simulink model "NonLinearModelWithObserver_real"  (R2022a)
settings: Solver=FixedStepAuto  StartTime=0.0  StopTime=inf  FixedStep=0.01  MaxStep=1e-3  MinStep=1e-5  RelTol=1e-3  EnableMultiTasking=on
values from neighbouring files (symbols this model uses):
  A = A_lin    [parameter_values.m]
  B = B_lin    [parameter_values.m]
  C_obs = [1 0 0 0; 0 0 1 0]    [parameter_values.m]
  K_lmi = calc_LMI_Controller(A,B,3)    [parameter_values.m]
  L = inv(P_sol)*N_sol    [calc_LMI_Observer.m]    (also in parameter_values.m = calc_LMI_Observer(A,C_obs,10))
  x0 = [deg2rad(0.1); 0; 0; 0]    [parameter_values.m]
  x_hat_0 = [0 0 0 0]    [parameter_values.m]
libraries: simulink_extras x1, svdutilitieslib x1, mbedblockslib x1
settings Model: ExtModeTrigDuration=10  Creator=schulte  LastModifiedBy=adlipke
settings SolverCC: AlgebraicLoopSolver=TrustRegion
settings DataIOCC: ReturnWorkspaceOutputs=off
settings OptimizationCC: EnhancedBackFolding=on  PassReuseOutputArgsAs=Individual arguments  ZeroExternalMemoryAtStartup=off  ZeroInternalMemoryAtStartup=off  MaxStackSize=64  OptimizeBlockOrder=speed  DifferentSizesBufferReuse=on  OptimizationCustomize=off  EfficientTunableParamExpr=on
settings DebuggingCC: ParameterTunabilityLossMsg=error  UnconnectedInputMsg=warning  UnconnectedOutputMsg=warning  UnconnectedLineMsg=warning  SFUnexpectedBacktrackingDiag=warning  SFNoUnconditionalDefaultTransitionDiag=warning  SFMachineParentedDataDiag=warning  ArithmeticOperatorsInVariantConditions=warning
settings HardwareCC: ProdBitPerPointer=32  ProdBitPerSizeT=32  ProdBitPerPtrDiffT=32  ProdLargestAtomicInteger=Long  ProdLargestAtomicFloat=Double  ProdWordSize=32  ProdLongLongMode=on  ProdHWDeviceType=ARM Compatible->ARM Cortex
settings SFSimCC: SimUseLocalCustomCode=off  MATLABDynamicMemAlloc=off  CustomCodeUndefinedFunction=UseInterfaceOnly
settings RTWCC: SystemTargetFile=ert.tlc  HardwareBoard=STM32 Nucleo L476RG  TemplateMakefile=ert_default_tmf  RTWUseLocalCustomCode=off  Toolchain=GNU Tools for ARM Embedded Processors
settings CodeAppCC: ForceParamTrailComments=on  IgnoreCustomStorageClasses=off  OperatorAnnotations=on  SimulinkDataObjDesc=on  SFDataObjDesc=on  InsertBlockDesc=on
settings ERTTargetCC: SupportContinuousTime=on  ExtModeTransport=3  ExtModeStaticAlloc=on  ExtModeStaticAllocSize=2000  ExtModeMexFile=ext_xcp  ExtModeIntrfLevel=Level2 - Open
settings ConfigComp: CovMetricSettings=dw  CovSaveCumulativeToWorkspaceVar=on  CovSaveSingleToWorkspaceVar=on  CovExternalEMLEnable=off

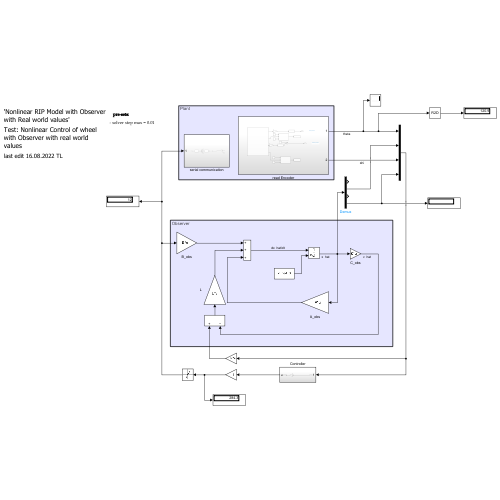
[thumbnail: Simulink's stored preview of the top-level diagram]
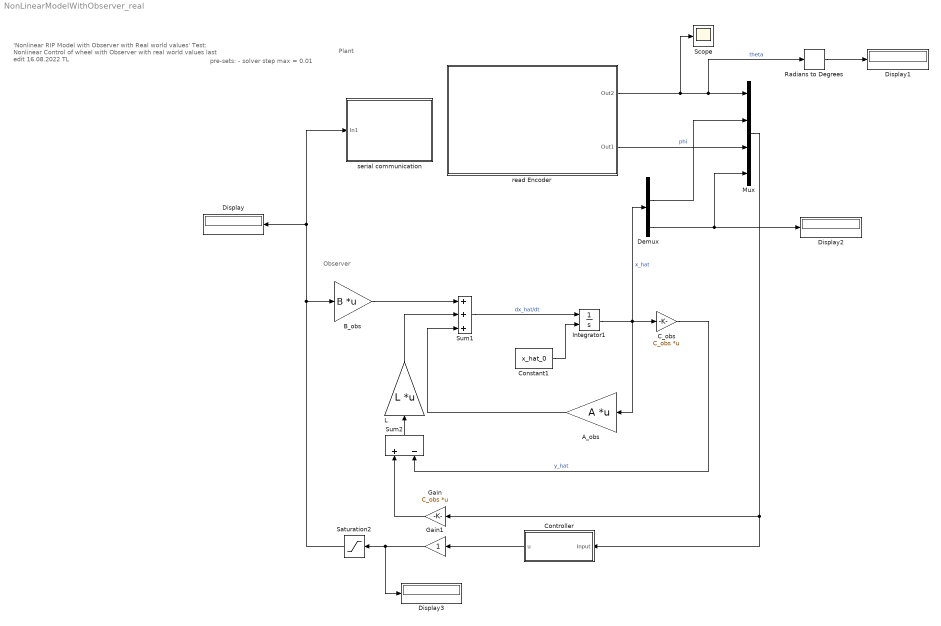
== system NonLinearModelWithObserver_real ==
  note: Plant
  note: Observer
  note: pre-sets:
      |
      | - solver step max = 0.01
  note: 'Nonlinear RIP Model with Observer with Real world values'
      |
      | Test: Nonlinear Control of wheel with Observer with real world values
      |
      | last edit 16.08.2022 TL
  A_obs : Gain  Gain=A  Multiplication=Matrix(K*u)
  B_obs : Gain  Gain=B  Multiplication=Matrix(K*u)
  C_obs : Gain  Gain=C_obs  Multiplication=Matrix(K*u)
  Constant1 : Constant  Value=x_hat_0
  Controller : Subsystem
  Demux : Demux
  Display{,1..3} (4 alike) : Display
  Gain : Gain  Gain=C_obs  Multiplication=Matrix(K*u)
  Gain1 : Gain
  Integrator1 : Integrator  InitialConditionSource=external  InitialCondition=x0
  L : Gain  Gain=L  Multiplication=Matrix(K*u)
  Mux : Mux
  Radians to Degrees : simulink_extras/Transformations/Radians to Degrees
  Saturation2 : Saturate  UpperLimit=12  LowerLimit=-12
  Scope : Scope
  Sum1 : Sum  Inputs=+++
  Sum2 : Sum  Inputs=+-
  read Encoder : Subsystem
  serial communication : Subsystem
  wires:
  A_obs/1 -> Sum1/3
  Sum2/1 -> L/1
  L/1 -> Sum1/2
  Sum1/1 -> Integrator1/1  "dx_hat/dt"
  C_obs/1 -> Sum2/2  "y_hat"
  B_obs/1 -> Sum1/1
  Constant1/1 -> Integrator1/2
  Integrator1/1 -> Demux/1, A_obs/1, C_obs/1  "x_hat"
  Controller/1(u) -> Gain1/1
  Demux/2 -> Mux/2
  Demux/4 -> Display2/1, Mux/4
  Mux/1 -> Controller/1(Input), Gain/1
  Gain/1 -> Sum2/1
  Saturation2/1 -> serial communication/1(In1), Display/1, B_obs/1
  read Encoder/2(Out1) -> Mux/3  "phi"
  read Encoder/1(Out2) -> Scope/1, Radians to Degrees/1, Mux/1  "theta"
  Gain1/1 -> Display3/1, Saturation2/1
  Radians to Degrees/1 -> Display1/1

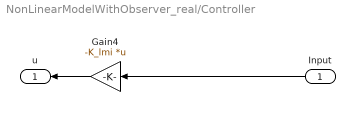
== system NonLinearModelWithObserver_real/Controller ==
  Input : Inport
  Gain4 : Gain  Gain=-K_lmi  Multiplication=Matrix(K*u)
  u : Outport
  wires:
  Gain4/1 -> u/1
  Input/1 -> Gain4/1

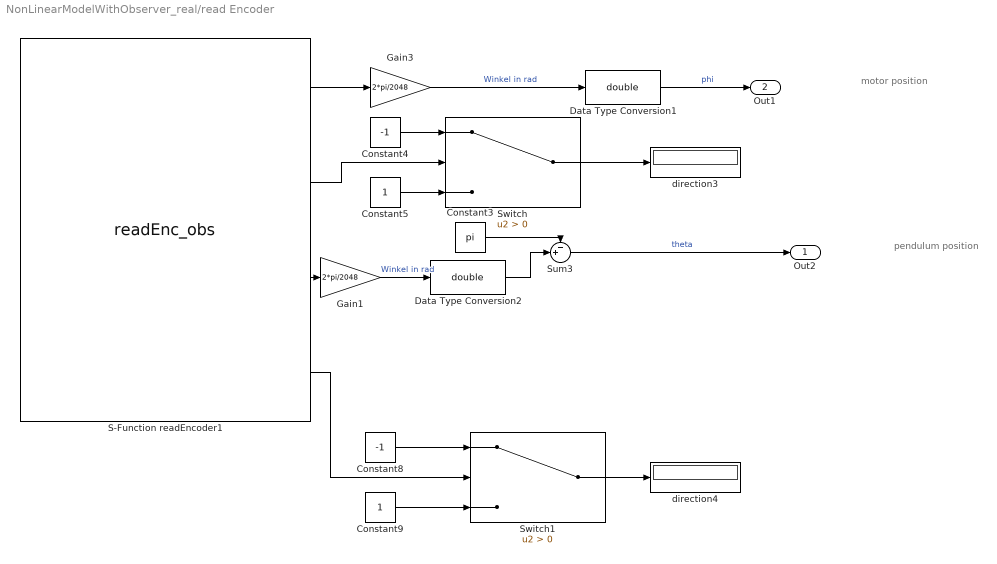
== system NonLinearModelWithObserver_real/read Encoder ==
  note: motor position
  note: pendulum position
  Constant3 : Constant  Value=pi
  Constant4 : Constant  Value=-1
  Constant5 : Constant
  Constant8 : Constant  Value=-1
  Constant9 : Constant
  Data Type Conversion1 : DataTypeConversion  OutDataTypeStr=double  SaturateOnIntegerOverflow=off  RndMeth=Floor
  Data Type Conversion2 : DataTypeConversion  OutDataTypeStr=double  SaturateOnIntegerOverflow=off  RndMeth=Floor
  Gain1 : Gain  Gain=2*pi/2048
  Gain3 : Gain  Gain=2*pi/2048
  S-Function readEncoder1 : S-Function  FunctionName=readEnc_obs  SFunctionModules=readEnc_obs_wrapper  SFunctionDeploymentMode=off  EnableBusSupport=off  mask(S-Function Builder){}
      mask help: Simulink:masks:SFunctionBuilder_MD
      mask init:
      | val = [[.9  0.75 0.75 1 1 .9 .9 1]',[1 1 0.75 0.75 .9 .9 1 .9]'];try , sys = get_param(gcb,'SfunBuilderFcnName');if isempty(sys), sys = get_param(gcb,'FunctionName'); end,catch, sys = get_param(gcb,'FunctionName'); end
      settings: CopyFcn=set_param(gcbh,'LinkStatus','none')  OpenFcn=sfunctionwizard(gcbh)
      mask Display:
      | plot(val(:,1),val(:,2))
      | disp(sys)
      | port_label('output',1,'tim2_cnt')
      | port_label('output',2,'tim2_dir')
      | port_label('output',3,'tim3_cnt')
      | port_label('output',4,'tim3_dir')
  Sum3 : Sum  Inputs=-+|
  Switch : Switch  Criteria=u2 > Threshold  SaturateOnIntegerOverflow=off  InputSameDT=off
  Switch1 : Switch  Criteria=u2 > Threshold  SaturateOnIntegerOverflow=off  InputSameDT=off
  direction3 : Display
  direction4 : Display
  Out2 : Outport
  Out1 : Outport  Port=2
  wires:
  Constant4/1 -> Switch/1
  Constant5/1 -> Switch/3
  S-Function readEncoder1/1 -> Gain3/1
  S-Function readEncoder1/4 -> Switch1/2
  Switch1/1 -> direction4/1
  S-Function readEncoder1/3 -> Gain1/1
  Constant8/1 -> Switch1/1
  Constant9/1 -> Switch1/3
  Gain3/1 -> Data Type Conversion1/1  "Winkel in rad"
  Data Type Conversion2/1 -> Sum3/2
  Switch/1 -> direction3/1
  Gain1/1 -> Data Type Conversion2/1  "Winkel in rad"
  Constant3/1 -> Sum3/1
  S-Function readEncoder1/2 -> Switch/2
  Sum3/1 -> Out2/1  "theta"
  Data Type Conversion1/1 -> Out1/1  "phi"

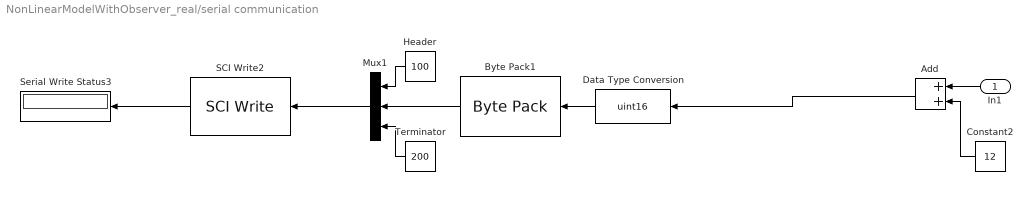
== system NonLinearModelWithObserver_real/serial communication ==
  In1 : Inport
  Add : Sum  AccumDataTypeStr=uint16  OutDataTypeStr=uint16
  Byte Pack1 : svdutilitieslib/Byte Pack  maskPackedDataType=uint8  datatypes={'uint16'}  byteAlign=1  blockPlatform=arduinoert
      settings: SourceProductBaseCode=ANDROID,ARDUINO,ML_ARDUINO,ECCORTEXA,ECCORTEXR,SC_BEAGLEBONE_BLUE,EC_FREEDOM_BOARD,EC_FRDM_K64F,INTEL_BLOCKSET,MICROBIT,NUCLEO,NVIDIA,PX4AUTOPILOTS,RASPPIIO,STMICRODIS,TIC2000,XILINX_BLOCKSET
  Constant2 : Constant  Value=12  OutDataTypeStr=single
  Data Type Conversion : DataTypeConversion  OutDataTypeStr=uint16  SaturateOnIntegerOverflow=off  RndMeth=Floor
  Header : Constant  Value=100  OutDataTypeStr=uint8  SampleTime=0.01
  Mux1 : Mux  Inputs=3
  SCI Write2 : mbedblockslib/SCI Write  SCIModule=1  Baudrate=uint32(9600)  Parity=None  StopBits=1  HardwareFlowControl=None  ByteOrder=LittleEndian  OutputStatus=on
      settings: SourceProductBaseCode=MICROBIT,NUCLEO,STMICRODIS
  Serial Write Status3 : Display
  Terminator : Constant  Value=200  OutDataTypeStr=uint8  SampleTime=0.01
  wires:
  Mux1/1 -> SCI Write2/1
  Terminator/1 -> Mux1/3
  Byte Pack1/1 -> Mux1/2
  Add/1 -> Data Type Conversion/1
  Data Type Conversion/1 -> Byte Pack1/1
  SCI Write2/1 -> Serial Write Status3/1
  Header/1 -> Mux1/1
  Constant2/1 -> Add/2
  In1/1 -> Add/1
